simulink model "Exp1_pendulum_validation"  (R2023b)
settings: Solver=ode3  StartTime=0.0  StopTime=Time(end)  FixedStep=0.001  RelTol=1e-3
undefined symbols (not defined in the file): Fgl, J, omega_0, phi_0, z
settings Model: Creator=tunkarlu  LastModifiedBy=tunkarlu

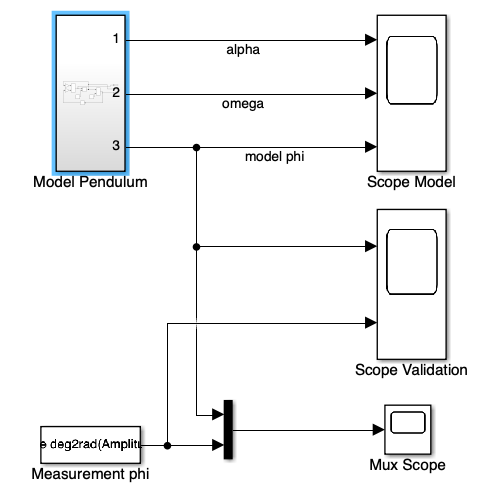
[thumbnail: Simulink's stored preview of the top-level diagram]
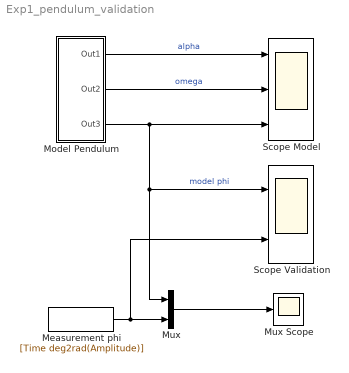
== system Exp1_pendulum_validation ==
  Measurement phi : FromWorkspace  VariableName=[Time deg2rad(Amplitude)]
  Model Pendulum : Subsystem
  Mux : Mux  Inputs=2
  Mux Scope : Scope
  Scope Model : Scope  NumInputPorts=3
  Scope Validation : Scope  NumInputPorts=2
  wires:
  Model Pendulum/1(Out1) -> Scope Model/1  "alpha"
  Model Pendulum/2(Out2) -> Scope Model/2  "omega"
  Model Pendulum/3(Out3) -> Scope Model/3, Scope Validation/1, Mux/1  "model phi"
  Mux/1 -> Mux Scope/1
  Measurement phi/1 -> Scope Validation/2, Mux/2

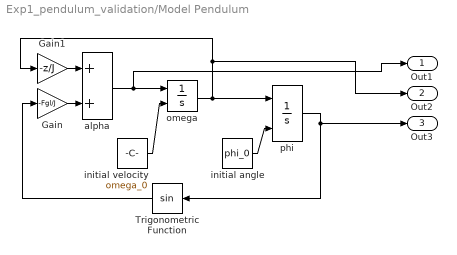
== system Exp1_pendulum_validation/Model Pendulum ==
  Gain : Gain  Gain=-Fgl/J
  Gain1 : Gain  Gain=-z/J
  Trigonometric Function : Trigonometry
  alpha : Sum
  initial angle : Constant  Value=phi_0
  initial velocity : Constant  Value=omega_0
  omega : Integrator  InitialConditionSource=external
  phi : Integrator  InitialConditionSource=external
  Out1 : Outport
  Out2 : Outport  Port=2
  Out3 : Outport  Port=3
  wires:
  Gain/1 -> alpha/2
  Trigonometric Function/1 -> Gain/1
  alpha/1 -> Out1/1, omega/1
  initial velocity/1 -> omega/2
  Gain1/1 -> alpha/1
  initial angle/1 -> phi/2
  phi/1 -> Out3/1, Trigonometric Function/1
  omega/1 -> Gain1/1, Out2/1, phi/1
